simulink model "BATTERIE"  (R2024a)
settings: Solver=VariableStepAuto  StartTime=0.0  StopTime=3600  RelTol=1e-3
settings Model: Creator=emanuele  LastModifiedBy=emanuele

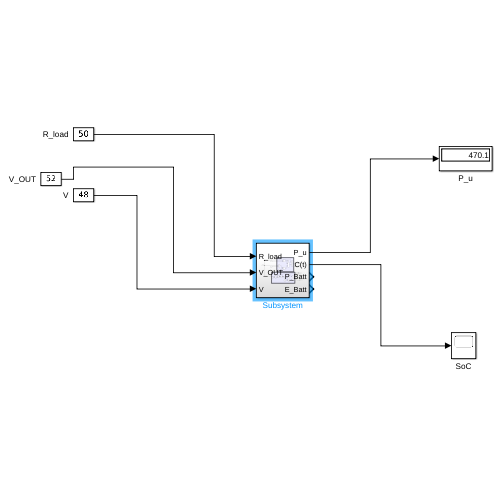
[thumbnail: Simulink's stored preview of the top-level diagram]
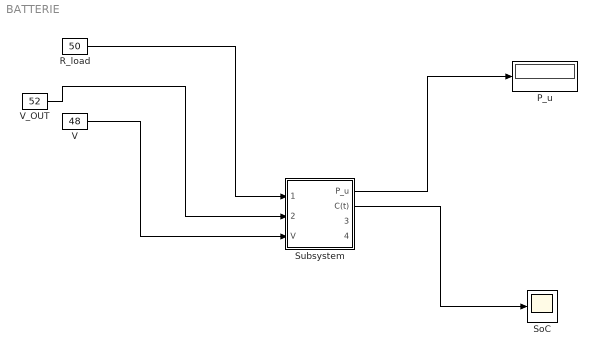
== system BATTERIE ==
  P_u : Display
  R_load : Constant  Value=50
  SoC : Scope
  Subsystem : Subsystem
  V : Constant  Value=48
  V_OUT : Constant  Value=52
  wires:
  R_load/1 -> Subsystem/1(R_load)
  V_OUT/1 -> Subsystem/2(V_OUT)
  V/1 -> Subsystem/3(V)
  Subsystem/1(P_u) -> P_u/1
  Subsystem/2(C(t)) -> SoC/1

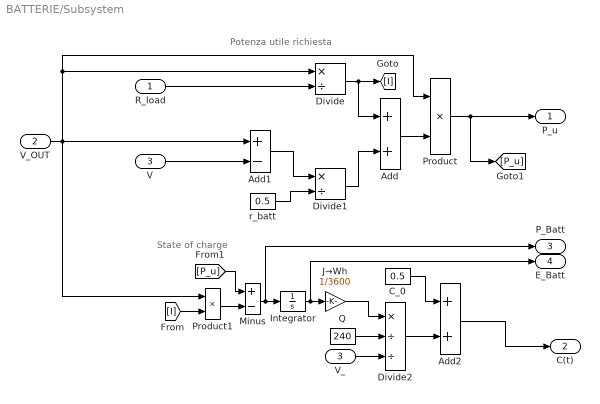
== system BATTERIE/Subsystem ==
  note: State of charge
  note: Potenza utile richiesta
  R_load : Inport
  V_OUT : Inport  Port=2
  V : Inport  Port=3
  Add : Sum
  Add1 : Sum  Inputs=+-
  Add2 : Sum
  C_0 : Constant  Value=0.5
  Divide : Product  Inputs=*/
  Divide1 : Product  Inputs=*/
  Divide2 : Product  Inputs=*//
  Integrator : Integrator
  J→Wh : Gain  Gain=1/3600
  Minus : Sum  Inputs=+-
  Product : Product
  Product1 : Product
  Q : Constant  Value=240
  V_ : InportShadow  Port=3
  r_batt : Constant  Value=0.5
  P_u : Outport
  C(t) : Outport  Port=2
  P_Batt : Outport  Port=3
  E_Batt : Outport  Port=4
  wires:
  V/1 -> Add1/2
  C_0/1 -> Add2/1
  Divide1/1 -> Add/2
  Integrator/1 -> E_Batt/1, J→Wh/1
  r_batt/1 -> Divide1/2
  V_OUT/1 -> Add1/1, Divide/1, Product/1, Product1/1
  Add1/1 -> Divide1/1
  Divide2/1 -> Add2/2
  Product1/1 -> Minus/2
  Add2/1 -> C(t)/1
  Add/1 -> Product/2
  Divide/1 -> [I], Add/1
  R_load/1 -> Divide/2
  Product/1 -> [P_u], P_u/1
  J→Wh/1 -> Divide2/1
  [I] -> Product1/2
  Minus/1 -> P_Batt/1, Integrator/1
  Q/1 -> Divide2/2
  [P_u] -> Minus/1
  V_/1 -> Divide2/3
